simulink model "Test_GSM_ZP_Tabelle"  (R2017b)
settings: Solver=VariableStepAuto  StartTime=0.0  StopTime=Inf  RelTol=1e-3
settings Model: Creator=张紫薇  LastModifiedBy=张紫薇

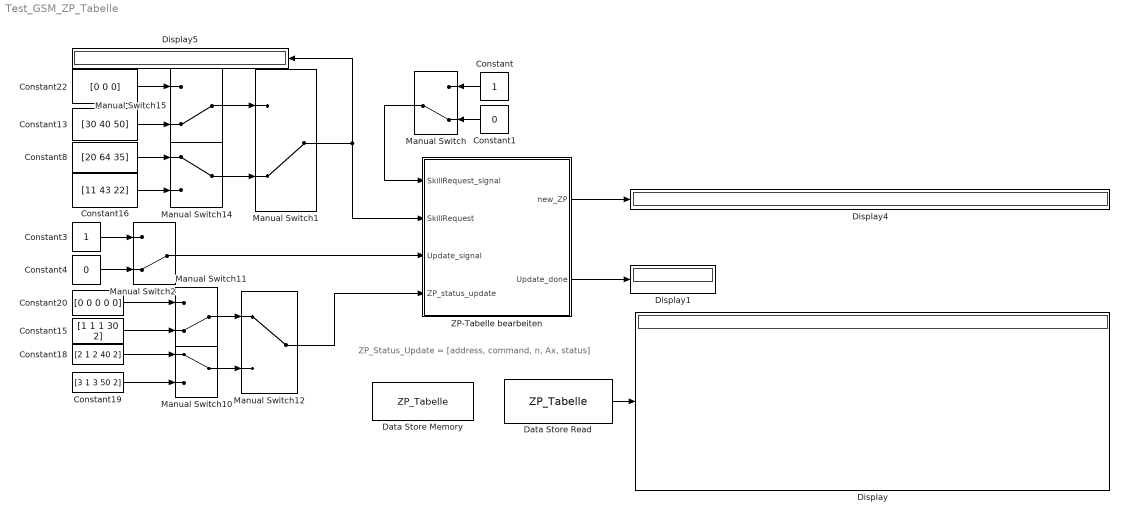
== system Test_GSM_ZP_Tabelle ==
  note: ZP_Status_Update = [address, command, n, Ax, status]
  Constant : Constant
  Constant1 : Constant  Value=0
  Constant13 : Constant  Value=[30 40 50]
  Constant15 : Constant  Value=[1 1 1 30 2]
  Constant16 : Constant  Value=[11 43 22]
  Constant18 : Constant  Value=[2 1 2 40 2]
  Constant19 : Constant  Value=[3 1 3 50 2]
  Constant20 : Constant  Value=[0 0 0 0 0]
  Constant22 : Constant  Value=[0 0 0]
  Constant3 : Constant
  Constant4 : Constant  Value=0
  Constant8 : Constant  Value=[20 64 35]
  Data Store Memory : DataStoreMemory  DataStoreName=ZP_Tabelle  ReadBeforeWriteMsg=warning  WriteAfterWriteMsg=warning  WriteAfterReadMsg=warning  InitialValue=zeros(10,7)  ShowAdditionalParam=off  OutDataTypeStr=double  Dimensions=[10 7]
  Data Store Read : DataStoreRead  DataStoreName=ZP_Tabelle
  Display{,1,4..5} (4 alike) : Display
  Manual Switch{,1..2,11,15} (5 alike) : ManualSwitch  CurrentSetting=0
  Manual Switch10 : ManualSwitch
  Manual Switch12 : ManualSwitch
  Manual Switch14 : ManualSwitch
  ZP-Tabelle bearbeiten : Subsystem
  wires:
  ZP-Tabelle bearbeiten/1(new_ZP) -> Display4/1
  Constant/1 -> Manual Switch/1
  Constant1/1 -> Manual Switch/2
  Manual Switch/1 -> ZP-Tabelle bearbeiten/1(SkillRequest_signal)
  Manual Switch15/1 -> Manual Switch1/1
  Manual Switch14/1 -> Manual Switch1/2
  Constant16/1 -> Manual Switch14/2
  Constant8/1 -> Manual Switch14/1
  Constant13/1 -> Manual Switch15/2
  Constant22/1 -> Manual Switch15/1
  Manual Switch1/1 -> Display5/1, ZP-Tabelle bearbeiten/2(SkillRequest)
  Constant4/1 -> Manual Switch2/2
  Constant3/1 -> Manual Switch2/1
  Manual Switch2/1 -> ZP-Tabelle bearbeiten/3(Update_signal)
  ZP-Tabelle bearbeiten/2(Update_done) -> Display1/1
  Constant18/1 -> Manual Switch10/1
  Constant15/1 -> Manual Switch11/2
  Constant20/1 -> Manual Switch11/1
  Manual Switch11/1 -> Manual Switch12/1
  Manual Switch10/1 -> Manual Switch12/2
  Constant19/1 -> Manual Switch10/2
  Manual Switch12/1 -> ZP-Tabelle bearbeiten/4(ZP_status_update)
  Data Store Read/1 -> Display/1

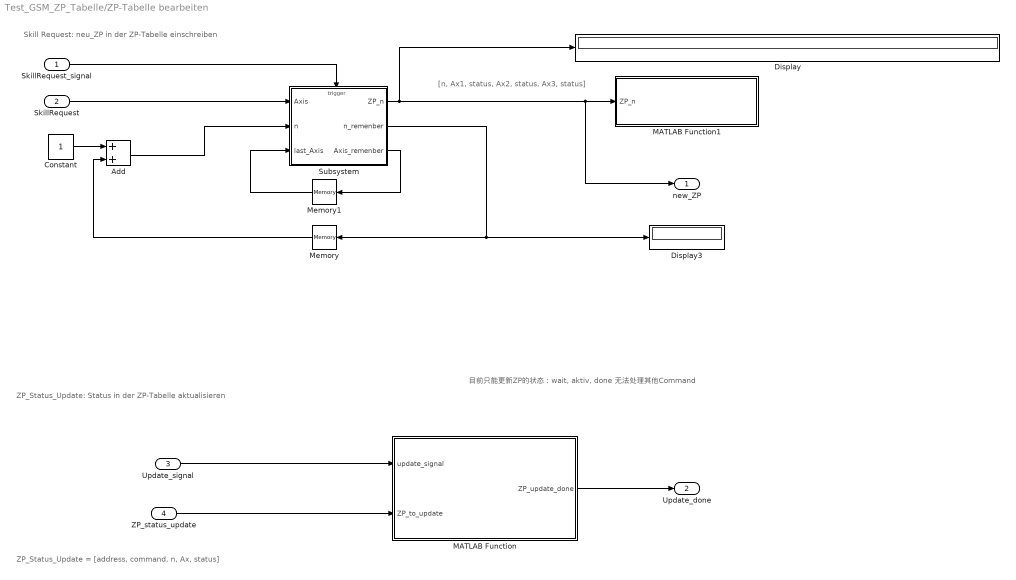
== system Test_GSM_ZP_Tabelle/ZP-Tabelle bearbeiten ==
  note: ZP_Status_Update = [address, command, n, Ax, status]
  note: Skill Request: neu_ZP in der ZP-Tabelle einschreiben
  note: 目前只能更新ZP的状态：wait, aktiv, done
      | 无法处理其他Command
  note: ZP_Status_Update: Status in der ZP-Tabelle aktualisieren
  note: [n, Ax1, status, Ax2, status, Ax3, status]
  SkillRequest_signal : Inport
  SkillRequest : Inport  Port=2
  Update_signal : Inport  Port=3
  ZP_status_update : Inport  Port=4  PortDimensions=5
  Add : Sum
  Constant : Constant
  Display : Display
  Display3 : Display
  MATLAB Function : MATLAB Function  TreatAsAtomicUnit=on
  MATLAB Function1 : MATLAB Function  TreatAsAtomicUnit=on
  Memory : Memory
  Memory1 : Memory  InitialCondition=[0 0 0]
  Subsystem : Subsystem
  new_ZP : Outport
  Update_done : Outport  Port=2
  wires:
  SkillRequest_signal/1 -> Subsystem/Trigger
  ZP_status_update/1 -> MATLAB Function/2(ZP_to_update)
  Subsystem/1(ZP_n) -> Display/1, MATLAB Function1/1(ZP_n), new_ZP/1
  MATLAB Function/1(ZP_update_done) -> Update_done/1
  Subsystem/2(n_remenber) -> Memory/1, Display3/1
  Constant/1 -> Add/1
  Add/1 -> Subsystem/2(n)
  Memory/1 -> Add/2
  Update_signal/1 -> MATLAB Function/1(update_signal)
  SkillRequest/1 -> Subsystem/1(Axis)
  Subsystem/3(Axis_remenber) -> Memory1/1
  Memory1/1 -> Subsystem/3(last_Axis)

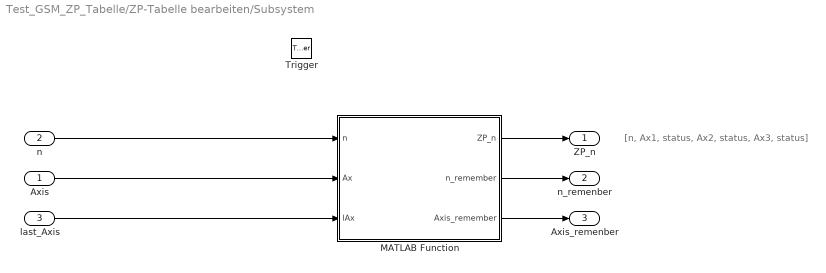
== system Test_GSM_ZP_Tabelle/ZP-Tabelle bearbeiten/Subsystem ==
  note: [n, Ax1, status, Ax2, status, Ax3, status]
  Axis : Inport
  n : Inport  Port=2
  last_Axis : Inport  Port=3
  Trigger : TriggerPort  VariantControl=Variant  PortDimensions=1
  MATLAB Function : MATLAB Function  TreatAsAtomicUnit=on
  ZP_n : Outport
  n_remenber : Outport  Port=2
  Axis_remenber : Outport  Port=3
  wires:
  n/1 -> MATLAB Function/1(n)
  Axis/1 -> MATLAB Function/2(Ax)
  MATLAB Function/1(ZP_n) -> ZP_n/1
  last_Axis/1 -> MATLAB Function/3(lAx)
  MATLAB Function/2(n_remember) -> n_remenber/1
  MATLAB Function/3(Axis_remember) -> Axis_remenber/1

== matlab function Test_GSM_ZP_Tabelle/ZP-Tabelle bearbeiten/Subsystem/MATLAB Function ==
  data: n input; ZP_n output; Ax input; lAx input; n_remember output; Axis_remember output
%ZP_n = [n, Ax1, status, Ax2, status, Ax3, status];

function [ZP_n, n_remember, Axis_remember] = Zielposition(n, Ax, lAx)

if ((Ax(1) == lAx(1)) && (Ax(2) == lAx(2)) && (Ax(3) == lAx(3))) == 0   %wiederholte Position filtern
    ZP_n = [n, Ax(1), 1, Ax(2), 1, Ax(3), 1];
    n_remember = n;
else
    ZP_n = [n-1, lAx(1), 1, lAx(2), 1, lAx(3),1];     %ZP_n ändert sich nicht
    n_remember = n-1;
end

Axis_remember = Ax;
end

== matlab function Test_GSM_ZP_Tabelle/ZP-Tabelle bearbeiten/MATLAB Function ==
  data: update_signal input; ZP_to_update input; ZP_update_done output; ZP_Tabelle data_store_memory
%ZP_Status_Update = [address, command, n, Ax, status]
%function [ZP_update_done, Update_Data] = Status_Update(update_signal, ZP_to_update, ZP_Tab)

function ZP_update_done  = Status_Update(update_signal, ZP_to_update)

global ZP_Tabelle

N=0;
m=0;
n=0;

if update_signal==1
    address = ZP_to_update(1);
    m = 2 * address + 1;
    n = ZP_to_update(3);
    status = ZP_to_update(5);
    
    for i=1:10
        if ZP_Tabelle(i,1) == n
            N = i;              %ZP_N bestimmen
            break
        end
    end
    
    %N==1, status aktualisieren
    %N>1 && (status von ZP_N-1 == 'done'), status aktualisieren
    if (N == 1) || (N>1 && (ZP_Tabelle(N-1,3) == ZP_Tabelle(N-1,5) == ZP_Tabelle(N-1,7) == 3))
        ZP_Tabelle(N,m) = status;
        ZP_update_done = 1;
    else        
        ZP_update_done = 0;
    end
else
    ZP_update_done = 0;
end

%Update_Data = ZP_Tabelle;

== matlab function Test_GSM_ZP_Tabelle/ZP-Tabelle bearbeiten/MATLAB Function1 ==
  data: ZP_n input; ZP_Tabelle data_store_memory
%ZP_n = [n, Ax1, status1, Ax2, status2, Ax3, status3];
%function ZP_newTable = new_ZP(ZP_n)

function new_ZP(ZP_n)

global ZP_Tabelle

m=0;
n = ZP_n(1);

for i = 1:10
    if ZP_Tabelle(i,1) == n
        break;
    end
    if ZP_Tabelle(i,1) == 0
        m=i;
        break
    end
end

if m ~= 0
    ZP_Tabelle(m,:) = ZP_n;
end

end
